simulink model "check_other_Potential"  (R2023b)
settings: Solver=ode5  StartTime=0.0  StopTime=2  FixedStep=0.0001  RelTol=1e-3
settings Model: Creator=amaiani  LastModifiedBy=amaiani

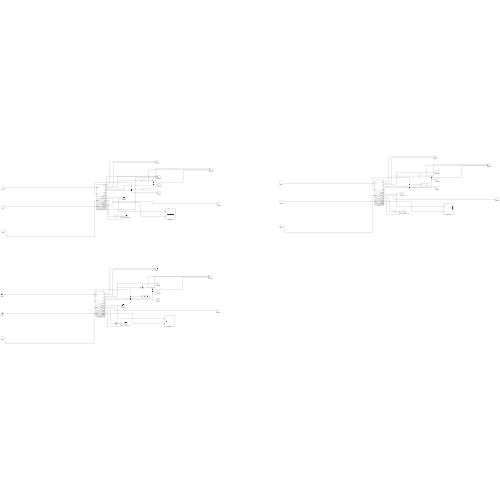
[thumbnail: Simulink's stored preview of the top-level diagram]
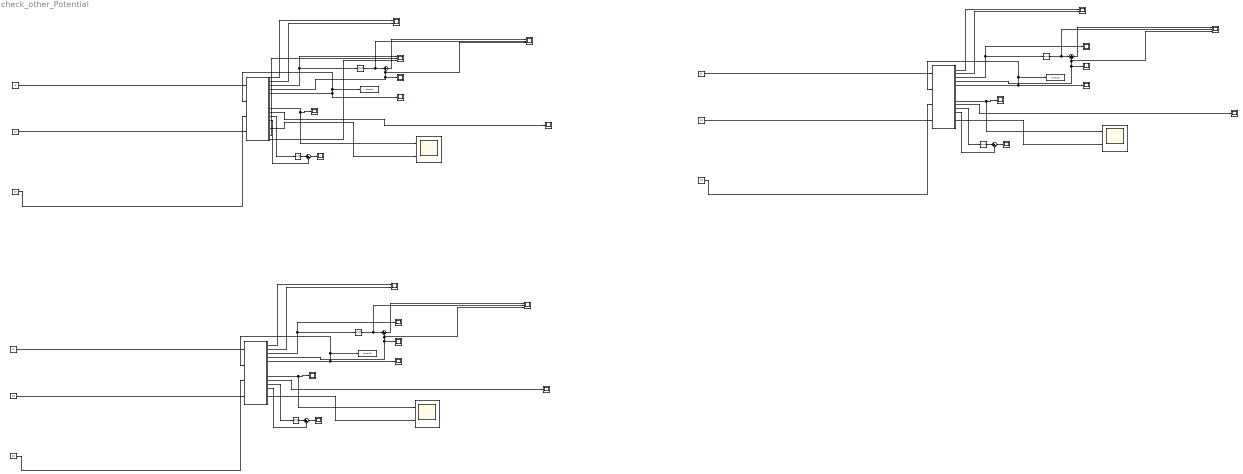
== system check_other_Potential ==
  Damp : Constant  Value=10
  Damp1 : Constant  Value=10
  Damp2 : Constant  Value=10
  Derivative{,1..5} (6 alike) : Derivative
  Dynamics{,1..5} (6 alike) : Scope
  H_dot_error : Scope  NumInputPorts=3
  H_dot_error1 : Scope  NumInputPorts=3
  H_dot_error2 : Scope  NumInputPorts=3
  H_dot_theory : Scope
  H_dot_theory1 : Scope
  H_dot_theory2 : Scope
  Hamiltonian : Scope  NumInputPorts=3
  Hamiltonian1 : Scope
  Hamiltonian2 : Scope
  Liu : Subsystem
  Liu1 : Subsystem
  Liu2 : Subsystem
  Sum{,1..5} (6 alike) : Sum  Inputs=|+-
  To Workspace : ToWorkspace  VariableName=simout  SampleTime=-1
  To Workspace1 : ToWorkspace  VariableName=simout1  SampleTime=-1
  To Workspace2 : ToWorkspace  VariableName=simout2  SampleTime=-1
  added_power : Scope  NumInputPorts=2
  added_power1 : Scope  NumInputPorts=2
  added_power2 : Scope  NumInputPorts=2
  alpha : Constant  Value=10
  alpha1 : Constant  Value=10
  alpha2 : Constant  Value=10
  cbf_dot_measured_error : Scope
  cbf_dot_measured_error1 : Scope
  cbf_dot_measured_error2 : Scope
  dhdqqdot : Scope
  dhdqqdot1 : Scope
  dhdqqdot2 : Scope
  skew : Scope  NumInputPorts=2
  skew1 : Scope  NumInputPorts=2
  skew2 : Scope  NumInputPorts=2
  spring : Constant  Value=[10,0,0;0,1,0;0,0,1]
  spring1 : Constant  Value=[10,0,0;0,10,0;0,0,10]
  spring2 : Constant  Value=[10,0,0;0,1,0;0,0,1]
  wires:
  Derivative/1 -> H_dot_error/2, Sum/1
  Sum/1 -> H_dot_error/1
  spring/1 -> Liu/1(spring)
  Damp/1 -> Liu/4(damp)
  alpha/1 -> Liu/3(alpha)
  Liu/4(H_dot) -> H_dot_theory/1, H_dot_error/3, Sum/2
  Liu/5(Out5) -> Dynamics/1, Liu/2(q), To Workspace/1
  Liu/3(E) -> Derivative/1, Hamiltonian/1
  Liu/1(out_1) -> skew/1
  Liu/2(out_2) -> skew/2
  Liu/10(hessian_term) -> Dynamics1/1
  Liu/9(before_dot) -> added_power/1, dhdqqdot/1
  Liu/11(cbf) -> Derivative1/1
  Derivative1/1 -> Sum2/1
  Sum2/1 -> cbf_dot_measured_error/1
  Liu/12(cbf_dot) -> Sum2/2
  Liu/14(after_dot) -> added_power/2
  Damp1/1 -> Liu1/4(damp)
  Liu1/2(out_2) -> skew1/2
  Liu1/11(cbf) -> Derivative3/1
  spring1/1 -> Liu1/1(spring)
  alpha1/1 -> Liu1/3(alpha)
  Liu1/5(Out5) -> Dynamics2/1, Liu1/2(q), To Workspace1/1
  Sum3/1 -> cbf_dot_measured_error1/1
  Liu1/1(out_1) -> skew1/1
  Liu1/10(hessian_term) -> Dynamics3/1
  Derivative2/1 -> H_dot_error1/2, Sum1/1
  Liu1/3(E) -> Derivative2/1, Hamiltonian1/1
  Derivative3/1 -> Sum3/1
  Liu1/12(cbf_dot) -> Sum3/2
  Sum1/1 -> H_dot_error1/1
  Liu1/4(H_dot) -> H_dot_theory1/1, H_dot_error1/3, Sum1/2
  Liu1/14(after_dot) -> added_power1/2
  Liu1/9(before_dot) -> added_power1/1, dhdqqdot1/1
  Damp2/1 -> Liu2/4(damp)
  Liu2/2(out_2) -> skew2/2
  Liu2/11(cbf) -> Derivative5/1
  spring2/1 -> Liu2/1(spring)
  alpha2/1 -> Liu2/3(alpha)
  Liu2/5(Out5) -> Dynamics4/1, Liu2/2(q), To Workspace2/1
  Sum5/1 -> cbf_dot_measured_error2/1
  Liu2/1(out_1) -> skew2/1
  Liu2/10(hessian_term) -> Dynamics5/1
  Derivative4/1 -> H_dot_error2/2, Sum4/1
  Liu2/3(E) -> Derivative4/1, Hamiltonian2/1
  Derivative5/1 -> Sum5/1
  Liu2/12(cbf_dot) -> Sum5/2
  Sum4/1 -> H_dot_error2/1
  Liu2/4(H_dot) -> H_dot_theory2/1, H_dot_error2/3, Sum4/2
  Liu2/14(after_dot) -> added_power2/2
  Liu2/9(before_dot) -> added_power2/1, dhdqqdot2/1
  Liu/16(T) -> Hamiltonian/2
  Liu/17(V) -> Hamiltonian/3

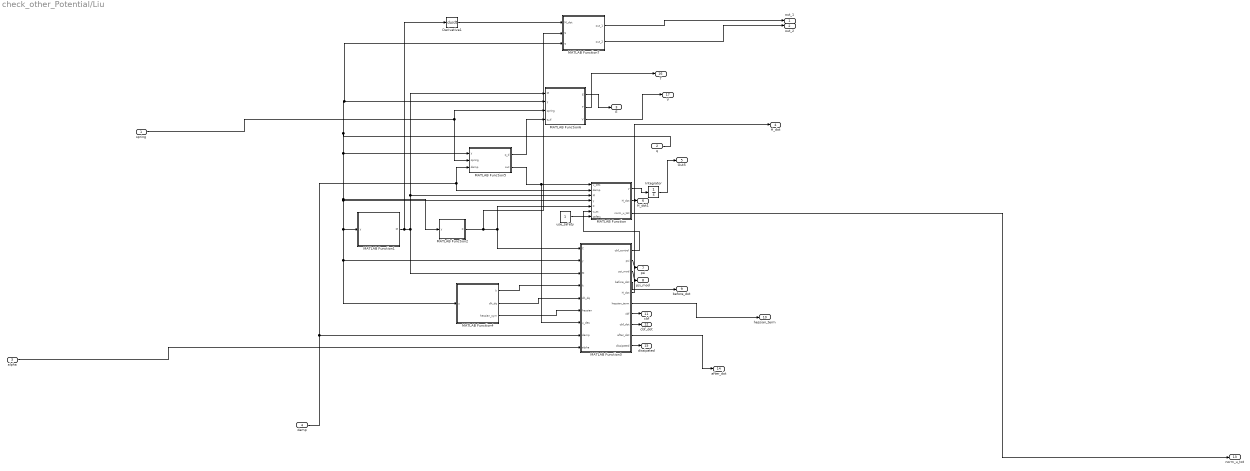
== system check_other_Potential/Liu ==
  spring : Inport
  q : Inport  Port=2
  alpha : Inport  Port=3
  damp : Inport  Port=4
  Derivative1 : Derivative
  Integrator : Integrator  InitialCondition=[0;0;0;0;0;0]
  MATLAB Function : MATLAB Function  TreatAsAtomicUnit=on
  MATLAB Function1 : MATLAB Function  StartFcn=|  TreatAsAtomicUnit=on
      | % Define numerical values for the parameters
      | xc = 2.5;
      | yc = 2;
      | r = 1;
      | gamma = 2;
      | alpha = 20;
      | 
      | 
      | m1 = 1;
      | m2 = 1;
      | m3 = 1;
      | 
      | 
      | l1 = 1;
      | l2 = 1;
      | l3 = 1;
  MATLAB Function2 : MATLAB Function  StartFcn=|  TreatAsAtomicUnit=on
      | % Define numerical values for the parameters
      | xc = 2.5;
      | yc = 2;
      | r = 1;
      | gamma = 2;
      | alpha = 20;
      | 
      | 
      | m1 = 1;
      | m2 = 1;
      | m3 = 1;
      | 
      | 
      | l1 = 1;
      | l2 = 1;
      | l3 = 1;
  MATLAB Function3 : MATLAB Function  TreatAsAtomicUnit=on
  MATLAB Function4 : MATLAB Function  TreatAsAtomicUnit=on
  MATLAB Function5 : MATLAB Function  TreatAsAtomicUnit=on
  MATLAB Function6 : MATLAB Function  TreatAsAtomicUnit=on
  MATLAB Function7 : MATLAB Function  StartFcn=|  TreatAsAtomicUnit=on
      | % Define numerical values for the parameters
      | xc = 2.5;
      | yc = 2;
      | r = 1;
      | gamma = 2;
      | alpha = 20;
      | 
      | 
      | m1 = 1;
      | m2 = 1;
      | m3 = 1;
      | 
      | 
      | l1 = 1;
      | l2 = 1;
      | l3 = 1;
  use_safety : Constant
  out_1 : Outport
  out_2 : Outport  Port=2
  E : Outport  Port=3
  H_dot : Outport  Port=4
  Out5 : Outport  Port=5
  H_dot1 : Outport  Port=6
  psi : Outport  Port=7
  psi_mod : Outport  Port=8
  before_dot : Outport  Port=9
  hessian_term : Outport  Port=10
  cbf : Outport  Port=11
  cbf_dot : Outport  Port=12
  norm_u_tot : Outport  Port=13
  after_dot : Outport  Port=14
  dissipated : Outport  Port=15
  T : Outport  Port=16
  V : Outport  Port=17
  wires:
  MATLAB Function3/8(cbf_dot) -> cbf_dot/1
  MATLAB Function3/2(psi) -> psi/1
  MATLAB Function3/7(cbf) -> cbf/1
  MATLAB Function/3(norm_u_tot) -> norm_u_tot/1
  MATLAB Function/2(H_dot) -> H_dot1/1
  Integrator/1 -> Out5/1
  MATLAB Function4/3(hessian_sym) -> MATLAB Function3/6(hessian)
  MATLAB Function1/1(M) -> Derivative1/1, MATLAB Function6/1(M), MATLAB Function/3(M), MATLAB Function3/3(M)
  MATLAB Function4/2(dh_dq) -> MATLAB Function3/5(dh_dq)
  MATLAB Function7/1(out_1) -> out_1/1
  alpha/1 -> MATLAB Function3/9(alpha)
  MATLAB Function6/1(E) -> E/1
  MATLAB Function3/3(psi_mod) -> psi_mod/1
  MATLAB Function7/2(out_2) -> out_2/1
  use_safety/1 -> MATLAB Function/7(safety)
  MATLAB Function3/4(before_dot) -> before_dot/1
  Derivative1/1 -> MATLAB Function7/1(M_dot)
  MATLAB Function5/1(q_d) -> MATLAB Function6/4(q_d)
  MATLAB Function3/5(H_dot) -> H_dot/1
  MATLAB Function/1(y) -> Integrator/1
  MATLAB Function3/1(cbf_control) -> MATLAB Function/6(u_sc)
  MATLAB Function2/1(C) -> MATLAB Function/5(C), MATLAB Function3/1(C), MATLAB Function7/2(S)
  MATLAB Function4/1(h) -> MATLAB Function3/4(h)
  spring/1 -> MATLAB Function6/3(spring), MATLAB Function5/2(spring)
  MATLAB Function5/2(out) -> MATLAB Function3/7(u_des), MATLAB Function/1(u_des)
  MATLAB Function3/6(hessian_term) -> hessian_term/1
  q/1 -> MATLAB Function7/3(q), MATLAB Function6/2(y), MATLAB Function5/1(y), MATLAB Function2/1(y), MATLAB Function4/1(y), MATLAB Function3/2(y), MATLAB Function1/1(y), MATLAB Function/4("y ")
  damp/1 -> MATLAB Function/2(damp), MATLAB Function5/3(damp), MATLAB Function3/8(damp)
  MATLAB Function3/9(after_dot) -> after_dot/1
  MATLAB Function3/10(dissipated) -> dissipated/1
  MATLAB Function6/2(T) -> T/1
  MATLAB Function6/3(V) -> V/1

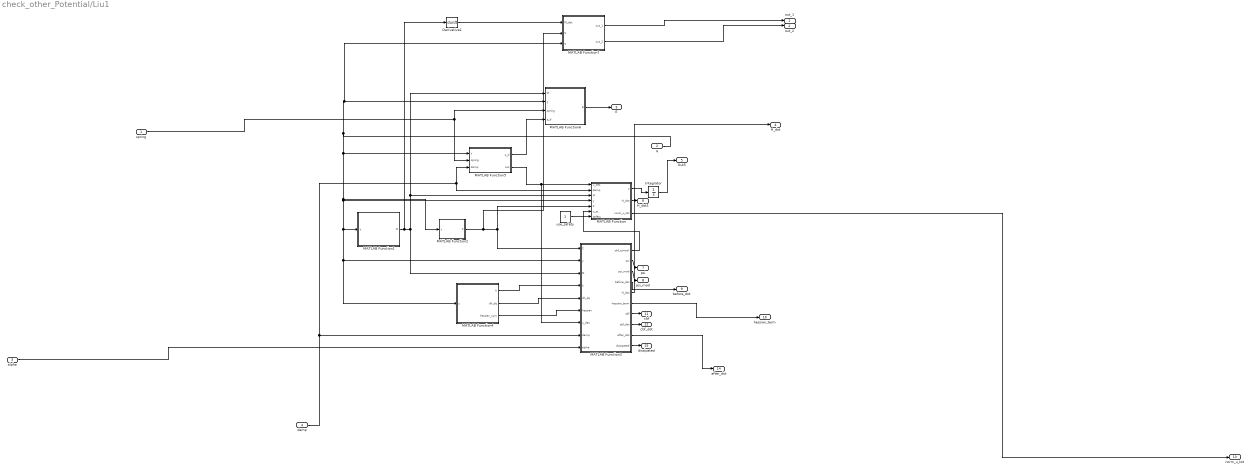
== system check_other_Potential/Liu1 ==
  spring : Inport
  q : Inport  Port=2
  alpha : Inport  Port=3
  damp : Inport  Port=4
  Derivative1 : Derivative
  Integrator : Integrator  InitialCondition=[0;0;0;0;0;0]
  MATLAB Function : MATLAB Function  TreatAsAtomicUnit=on
  MATLAB Function1 : MATLAB Function  StartFcn=|  TreatAsAtomicUnit=on
      | % Define numerical values for the parameters
      | xc = 2.5;
      | yc = 2;
      | r = 1;
      | gamma = 2;
      | alpha = 20;
      | 
      | 
      | m1 = 1;
      | m2 = 1;
      | m3 = 1;
      | 
      | 
      | l1 = 1;
      | l2 = 1;
      | l3 = 1;
  MATLAB Function2 : MATLAB Function  StartFcn=|  TreatAsAtomicUnit=on
      | % Define numerical values for the parameters
      | xc = 2.5;
      | yc = 2;
      | r = 1;
      | gamma = 2;
      | alpha = 20;
      | 
      | 
      | m1 = 1;
      | m2 = 1;
      | m3 = 1;
      | 
      | 
      | l1 = 1;
      | l2 = 1;
      | l3 = 1;
  MATLAB Function3 : MATLAB Function  TreatAsAtomicUnit=on
  MATLAB Function4 : MATLAB Function  TreatAsAtomicUnit=on
  MATLAB Function5 : MATLAB Function  TreatAsAtomicUnit=on
  MATLAB Function6 : MATLAB Function  TreatAsAtomicUnit=on
  MATLAB Function7 : MATLAB Function  StartFcn=|  TreatAsAtomicUnit=on
      | % Define numerical values for the parameters
      | xc = 2.5;
      | yc = 2;
      | r = 1;
      | gamma = 2;
      | alpha = 20;
      | 
      | 
      | m1 = 1;
      | m2 = 1;
      | m3 = 1;
      | 
      | 
      | l1 = 1;
      | l2 = 1;
      | l3 = 1;
  use_safety : Constant
  out_1 : Outport
  out_2 : Outport  Port=2
  E : Outport  Port=3
  H_dot : Outport  Port=4
  Out5 : Outport  Port=5
  H_dot1 : Outport  Port=6
  psi : Outport  Port=7
  psi_mod : Outport  Port=8
  before_dot : Outport  Port=9
  hessian_term : Outport  Port=10
  cbf : Outport  Port=11
  cbf_dot : Outport  Port=12
  norm_u_tot : Outport  Port=13
  after_dot : Outport  Port=14
  dissipated : Outport  Port=15
  wires:
  MATLAB Function3/8(cbf_dot) -> cbf_dot/1
  MATLAB Function3/2(psi) -> psi/1
  MATLAB Function3/7(cbf) -> cbf/1
  MATLAB Function/3(norm_u_tot) -> norm_u_tot/1
  MATLAB Function/2(H_dot) -> H_dot1/1
  Integrator/1 -> Out5/1
  MATLAB Function4/3(hessian_sym) -> MATLAB Function3/6(hessian)
  MATLAB Function1/1(M) -> Derivative1/1, MATLAB Function6/1(M), MATLAB Function/3(M), MATLAB Function3/3(M)
  MATLAB Function4/2(dh_dq) -> MATLAB Function3/5(dh_dq)
  MATLAB Function7/1(out_1) -> out_1/1
  alpha/1 -> MATLAB Function3/9(alpha)
  MATLAB Function6/1(E) -> E/1
  MATLAB Function3/3(psi_mod) -> psi_mod/1
  MATLAB Function7/2(out_2) -> out_2/1
  use_safety/1 -> MATLAB Function/7(safety)
  MATLAB Function3/4(before_dot) -> before_dot/1
  Derivative1/1 -> MATLAB Function7/1(M_dot)
  MATLAB Function5/1(q_d) -> MATLAB Function6/4(q_d)
  MATLAB Function3/5(H_dot) -> H_dot/1
  MATLAB Function/1(y) -> Integrator/1
  MATLAB Function3/1(cbf_control) -> MATLAB Function/6(u_sc)
  MATLAB Function2/1(C) -> MATLAB Function/5(C), MATLAB Function3/1(C), MATLAB Function7/2(S)
  MATLAB Function4/1(h) -> MATLAB Function3/4(h)
  spring/1 -> MATLAB Function6/3(spring), MATLAB Function5/2(spring)
  MATLAB Function5/2(out) -> MATLAB Function3/7(u_des), MATLAB Function/1(u_des)
  MATLAB Function3/6(hessian_term) -> hessian_term/1
  q/1 -> MATLAB Function7/3(q), MATLAB Function6/2(y), MATLAB Function5/1(y), MATLAB Function2/1(y), MATLAB Function4/1(y), MATLAB Function3/2(y), MATLAB Function1/1(y), MATLAB Function/4("y ")
  damp/1 -> MATLAB Function/2(damp), MATLAB Function5/3(damp), MATLAB Function3/8(damp)
  MATLAB Function3/9(after_dot) -> after_dot/1
  MATLAB Function3/10(dissipated) -> dissipated/1

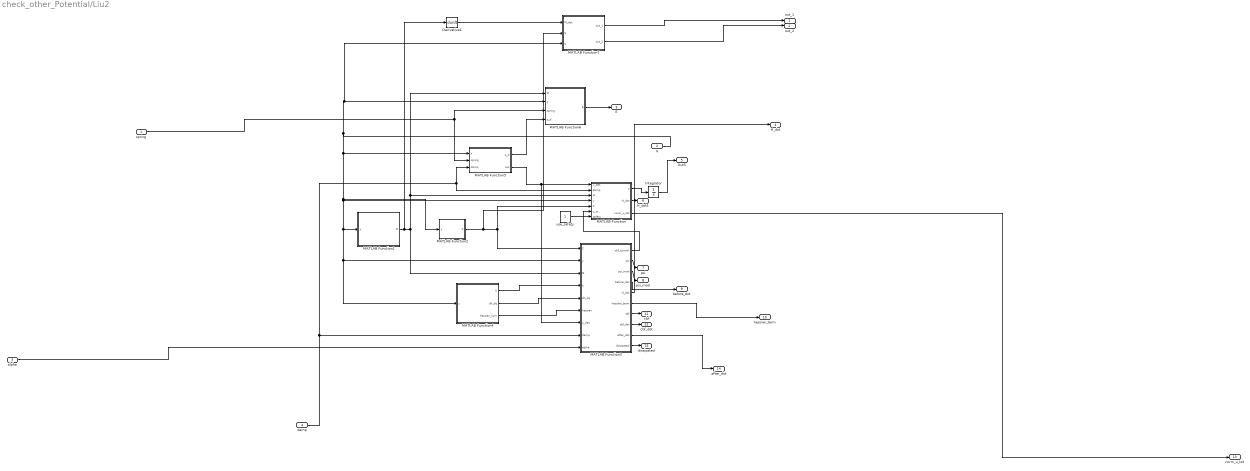
== system check_other_Potential/Liu2 ==
  spring : Inport
  q : Inport  Port=2
  alpha : Inport  Port=3
  damp : Inport  Port=4
  Derivative1 : Derivative
  Integrator : Integrator  InitialCondition=[0;0;0;0;0;0]
  MATLAB Function : MATLAB Function  TreatAsAtomicUnit=on
  MATLAB Function1 : MATLAB Function  StartFcn=|  TreatAsAtomicUnit=on
      | % Define numerical values for the parameters
      | xc = 2.5;
      | yc = 2;
      | r = 1;
      | gamma = 2;
      | alpha = 20;
      | 
      | 
      | m1 = 1;
      | m2 = 1;
      | m3 = 1;
      | 
      | 
      | l1 = 1;
      | l2 = 1;
      | l3 = 1;
  MATLAB Function2 : MATLAB Function  StartFcn=|  TreatAsAtomicUnit=on
      | % Define numerical values for the parameters
      | xc = 2.5;
      | yc = 2;
      | r = 1;
      | gamma = 2;
      | alpha = 20;
      | 
      | 
      | m1 = 1;
      | m2 = 1;
      | m3 = 1;
      | 
      | 
      | l1 = 1;
      | l2 = 1;
      | l3 = 1;
  MATLAB Function3 : MATLAB Function  TreatAsAtomicUnit=on
  MATLAB Function4 : MATLAB Function  TreatAsAtomicUnit=on
  MATLAB Function5 : MATLAB Function  TreatAsAtomicUnit=on
  MATLAB Function6 : MATLAB Function  TreatAsAtomicUnit=on
  MATLAB Function7 : MATLAB Function  StartFcn=|  TreatAsAtomicUnit=on
      | % Define numerical values for the parameters
      | xc = 2.5;
      | yc = 2;
      | r = 1;
      | gamma = 2;
      | alpha = 20;
      | 
      | 
      | m1 = 1;
      | m2 = 1;
      | m3 = 1;
      | 
      | 
      | l1 = 1;
      | l2 = 1;
      | l3 = 1;
  use_safety : Constant
  out_1 : Outport
  out_2 : Outport  Port=2
  E : Outport  Port=3
  H_dot : Outport  Port=4
  Out5 : Outport  Port=5
  H_dot1 : Outport  Port=6
  psi : Outport  Port=7
  psi_mod : Outport  Port=8
  before_dot : Outport  Port=9
  hessian_term : Outport  Port=10
  cbf : Outport  Port=11
  cbf_dot : Outport  Port=12
  norm_u_tot : Outport  Port=13
  after_dot : Outport  Port=14
  dissipated : Outport  Port=15
  wires:
  MATLAB Function3/8(cbf_dot) -> cbf_dot/1
  MATLAB Function3/2(psi) -> psi/1
  MATLAB Function3/7(cbf) -> cbf/1
  MATLAB Function/3(norm_u_tot) -> norm_u_tot/1
  MATLAB Function/2(H_dot) -> H_dot1/1
  Integrator/1 -> Out5/1
  MATLAB Function4/3(hessian_sym) -> MATLAB Function3/6(hessian)
  MATLAB Function1/1(M) -> Derivative1/1, MATLAB Function6/1(M), MATLAB Function/3(M), MATLAB Function3/3(M)
  MATLAB Function4/2(dh_dq) -> MATLAB Function3/5(dh_dq)
  MATLAB Function7/1(out_1) -> out_1/1
  alpha/1 -> MATLAB Function3/9(alpha)
  MATLAB Function6/1(E) -> E/1
  MATLAB Function3/3(psi_mod) -> psi_mod/1
  MATLAB Function7/2(out_2) -> out_2/1
  use_safety/1 -> MATLAB Function/7(safety)
  MATLAB Function3/4(before_dot) -> before_dot/1
  Derivative1/1 -> MATLAB Function7/1(M_dot)
  MATLAB Function5/1(q_d) -> MATLAB Function6/4(q_d)
  MATLAB Function3/5(H_dot) -> H_dot/1
  MATLAB Function/1(y) -> Integrator/1
  MATLAB Function3/1(cbf_control) -> MATLAB Function/6(u_sc)
  MATLAB Function2/1(C) -> MATLAB Function/5(C), MATLAB Function3/1(C), MATLAB Function7/2(S)
  MATLAB Function4/1(h) -> MATLAB Function3/4(h)
  spring/1 -> MATLAB Function6/3(spring), MATLAB Function5/2(spring)
  MATLAB Function5/2(out) -> MATLAB Function3/7(u_des), MATLAB Function/1(u_des)
  MATLAB Function3/6(hessian_term) -> hessian_term/1
  q/1 -> MATLAB Function7/3(q), MATLAB Function6/2(y), MATLAB Function5/1(y), MATLAB Function2/1(y), MATLAB Function4/1(y), MATLAB Function3/2(y), MATLAB Function1/1(y), MATLAB Function/4("y ")
  damp/1 -> MATLAB Function/2(damp), MATLAB Function5/3(damp), MATLAB Function3/8(damp)
  MATLAB Function3/9(after_dot) -> after_dot/1
  MATLAB Function3/10(dissipated) -> dissipated/1

== matlab function check_other_Potential/Liu/MATLAB Function6 ==
  data: M input; E output; y input; spring input; q_d input; T output; V output
function [E,T,V] = energy(M,y,spring, q_d)
    q = y(1:3);
    dq = y(4:6);
    T = 0.5 * (dq' * M * dq);
    V = 0.5 * (q-q_d)' *spring* (q-q_d);
    E = T + V;

== matlab function check_other_Potential/Liu/MATLAB Function7 ==
  data: M_dot input; out_1 output; S input; q input; out_2 output


function [out_1, out_2] = M_dot_coriolis_check(M_dot,S, q)
    dq = reshape(q(4:6),[3,1]);
    
    q1 = q(1);
    q2 = q(2);
    q3 = q(3);
    dq1 = q(4);
    dq2 = q(5);
    dq3 = q(6);

    check = M_dot - 2 * S;


    out_1 = dq' * check * dq;


    M_dot_formula =   [        - dq2*(sin(q2 + q3) + 3*sin(q2)) - dq3*(sin(q2 + q3) + sin(q3)), - dq3*(sin(q2 + q3)/2 + sin(q3)) - dq2*(sin(q2 + q3)/2 + (3*sin(q2))/2), - (dq2*sin(q2 + q3))/2 - dq3*(sin(q2 + q3)/2 + sin(q3)/2);
- dq3*(sin(q2 + q3)/2 + sin(q3)) - dq2*(sin(q2 + q3)/2 + (3*sin(q2))/2),                                                            -dq3*sin(q3),                                          -(dq3*sin(q3))/2;
              - (dq2*sin(q2 + q3))/2 - dq3*(sin(q2 + q3)/2 + sin(q3)/2),                                                        -(dq3*sin(q3))/2,                                                         0];
 

    
    out_2 = dq' * (M_dot_formula - 2 * S) * dq;
end

== matlab function check_other_Potential/Liu1/MATLAB Function ==
  data: u_des input; damp input; M input; y input; y output; C input; H_dot output; u_sc input; safety input; norm_u_tot output
function [y,H_dot,norm_u_tot]= dynamics(u_des, damp , M,y, C, u_sc, safety)
    
    q = reshape(y(1:3),[3,1]);
    dq = reshape(y(4:6),[3,1]);



    [~, p] = chol(M);
    decision = (p == 0);

    assert(decision, 'Inertia matrix is not positive definite');
    
    u_tot = u_des + safety * u_sc;
    norm_u_tot=norm(u_tot);
    ddq = inv(M) * (u_tot - C * dq ); % + u_sc

    H_dot = - dq' * damp * dq;

    y = [dq; ddq];

== matlab function check_other_Potential/Liu1/MATLAB Function1 ==
  data: y input; M output
function M = inertia_M(y)

    q1 = y(1);
    q2 = y(2);
    q3 = y(3);

    M  = [        cos(q2 + q3) + 3*cos(q2) + cos(q3) + 4, cos(q2 + q3)/2 + (3*cos(q2))/2 + cos(q3) + 5/3, cos(q2 + q3)/2 + cos(q3)/2 + 1/3;
cos(q2 + q3)/2 + (3*cos(q2))/2 + cos(q3) + 5/3,                                  cos(q3) + 5/3,                  cos(q3)/2 + 1/3;
              cos(q2 + q3)/2 + cos(q3)/2 + 1/3,                                cos(q3)/2 + 1/3,                              1/3];

    assert(isequal(M, M'),'error')

== matlab function check_other_Potential/Liu1/MATLAB Function2 ==
  data: y input; C output
function C = coriolis(y)

    q1 = y(1);
    q2 = y(2);
    q3 = y(3);
    dq1 = y(4);
    dq2 = y(5);
    dq3 = y(6);


    C = [- dq2*(sin(q2 + q3)/2 + (3*sin(q2))/2) - dq3*(sin(q2 + q3)/2 + sin(q3)/2), - dq1*(sin(q2 + q3)/2 + (3*sin(q2))/2) - dq2*(sin(q2 + q3)/2 + (3*sin(q2))/2) - dq3*(sin(q2 + q3)/2 + sin(q3)/2), - dq1*(sin(q2 + q3)/2 + sin(q3)/2) - dq2*(sin(q2 + q3)/2 + sin(q3)/2) - dq3*(sin(q2 + q3)/2 + sin(q3)/2);
                dq1*(sin(q2 + q3)/2 + (3*sin(q2))/2) - (dq3*sin(q3))/2,                                                                                                 -(dq3*sin(q3))/2,                                                    - (dq1*sin(q3))/2 - (dq2*sin(q3))/2 - (dq3*sin(q3))/2;
                       dq1*(sin(q2 + q3)/2 + sin(q3)/2) + (dq2*sin(q3))/2,                                                                                (dq1*sin(q3))/2 + (dq2*sin(q3))/2,                                                                                                        0];

== matlab function check_other_Potential/Liu1/MATLAB Function3 ==
  data: C input; y input; cbf_control output; M input; h input; dh_dq input; hessian input; u_des input; psi output; psi_mod output; before_dot output; H_dot output; damp input; hessian_term output; cbf output; cbf_dot output; alpha input; after_dot output; dissipated output

function [cbf_control, psi, psi_mod,before_dot, H_dot, hessian_term, cbf, cbf_dot, after_dot, dissipated]= CBF(C, y, M, h, dh_dq, hessian, u_des, damp, alpha)
% Define numerical values for the parameters
    xc = 2.5;
    yc = 2;
    r = 1;
    gamma = 2;

    
    m1 = 1;
    m2 = 1;
    m3 = 1;
    
    l1 = 1;
    l2 = 1;
    l3 = 1;
    
    q = reshape(y(1:3),[3,1]);
    dq = reshape(y(4:6),[3,1]);
    dh_dq = reshape(dh_dq,[1,3]);

    LIU = 1;

    M_inv = inv(M);

    before_dot = dh_dq * dq;
    after_dot = dh_dq * M_inv * dq;



    d = eig(M_inv);
    tol = 10^(-5);
    check = all(abs(M_inv - M_inv') < tol, 'all');
    assert(check,'error')
    % assert(isequal(M_inv, M_inv'),'error')

    assert(all(d>0),'error_m_inv')

    active = 0;

    if LIU == 1

    
        cbf = alpha * h + dh_dq * dq;
        lg_h = zeros(1,3);
        cbf_dot_prior = alpha .* dh_dq * dq + dq' * hessian * dq + dh_dq * (M_inv* (-C * dq + u_des));
        psi = cbf_dot_prior + gamma .* cbf;
        if psi<0
            lg_h = dh_dq * M_inv;
            
            cbf_control =  - lg_h' /(lg_h * lg_h')  .* psi;
            active = 1;
        else
            cbf_control = zeros(3,1);

        end
        cbf_dot = alpha .* dh_dq * dq + dq' * hessian * dq + dh_dq * M_inv* (-C * dq + u_des+ cbf_control);
        psi_mod = cbf_dot + gamma .* cbf;

        H_dot = dq' * cbf_control - dq' * damp * dq;
        
        dissipated= - dq' * damp * dq;

        hessian_term = dq' * hessian * dq;
        
    
    else
        KE = 0.5 * dq' * M * dq;
        cbf = alpha * h - KE;
        lg_h = zeros(1,3);
        cbf_dot_prior = alpha .* dh_dq * dq - dq' * M_inv * u_des;
        psi = cbf_dot_prior + gamma .* cbf;
        if psi<0
            lg_h = -dq';
            cbf_control =  dq /(dq'*dq)  .* psi;
        else
            cbf_control = zeros(3,1);
        end
        cbf_dot =  alpha .* dh_dq * dq - dq' * M_inv * (u_des+cbf_control) ;
        psi_mod = cbf_dot + gamma .* cbf;

        H_dot = dq' * cbf_control - dq' * damp * dq;


        hessian_term = 0;
 
        
    end
    
end

== matlab function check_other_Potential/Liu1/MATLAB Function4 ==
  data: y input; h output; dh_dq output; hessian_sym output
function [h, dh_dq, hessian_sym] = obstacle(y)
    % Define numerical values for the parameters
    xc = 2.5;
    yc = 2;
    r = 1;

    l1 = 1;
    l2 = 1;
    l3 = 1;
    
    % Compute the end-effector position using forward kinematics
    q1 = y(1);
    q2 = y(2);
    q3 = y(3);
    
    x_ee = l1 * cos(q1) + l2 * cos(q1 + q2) + l3 * cos(q1 + q2 + q3);
    y_ee = l1 * sin(q1) + l2 * sin(q1 + q2) + l3 * sin(q1 + q2 + q3);
    
    % Compute the control barrier function h
    h = (xc - x_ee)^2 + (yc - y_ee)^2 - r^2;
    
    % Define the expressions for dh_dq and hessian_sym
    dh_dq = [2*(cos(q1 + q2 + q3) + cos(q1 + q2) + cos(q1))*(sin(q1 + q2 + q3) + sin(q1 + q2) + sin(q1) - 2) - 2*(sin(q1 + q2 + q3) + sin(q1 + q2) + sin(q1))*(cos(q1 + q2 + q3) + cos(q1 + q2) + cos(q1) - 5/2), 2*(cos(q1 + q2 + q3) + cos(q1 + q2))*(sin(q1 + q2 + q3) + sin(q1 + q2) + sin(q1) - 2) - 2*(sin(q1 + q2 + q3) + sin(q1 + q2))*(cos(q1 + q2 + q3) + cos(q1 + q2) + cos(q1) - 5/2), 2*cos(q1 + q2 + q3)*(sin(q1 + q2 + q3) + sin(q1 + q2) + sin(q1) - 2) - 2*sin(q1 + q2 + q3)*(cos(q1 + q2 + q3) + cos(q1 + q2) + cos(q1) - 5/2)];


    hessian_sym = [                                              2*(cos(q1 + q2 + q3) + cos(q1 + q2) + cos(q1))^2 - 2*(cos(q1 + q2 + q3) + cos(q1 + q2) + cos(q1))*(cos(q1 + q2 + q3) + cos(q1 + q2) + cos(q1) - 5/2) + 2*(sin(q1 + q2 + q3) + sin(q1 + q2) + sin(q1))^2 - 2*(sin(q1 + q2 + q3) + sin(q1 + q2) + sin(q1))*(sin(q1 + q2 + q3) + sin(q1 + q2) + sin(q1) - 2), 2*(cos(q1 + q2 + q3) + cos(q1 + q2))*(cos(q1 + q2 + q3) + cos(q1 + q2) + cos(q1)) - 2*(cos(q1 + q2 + q3) + cos(q1 + q2))*(cos(q1 + q2 + q3) + cos(q1 + q2) + cos(q1) - 5/2) + 2*(sin(q1 + q2 + q3) + sin(q1 + q2))*(sin(q1 + q2 + q3) + sin(q1 + q2) + sin(q1)) - 2*(sin(q1 + q2 + q3) + sin(q1 + q2))*(sin(q1 + q2 + q3) + sin(q1 + q2) + sin(q1) - 2), 2*cos(q1 + q2 + q3)*(cos(q1 + q2 + q3) + cos(q1 + q2) + cos(q1)) - 2*cos(q1 + q2 + q3)*(cos(q1 + q2 + q3) + cos(q1 + q2) + cos(q1) - 5/2) + 2*sin(q1 + q2 + q3)*(sin(q1 + q2 + q3) + sin(q1 + q2) + sin(q1)) - 2*sin(q1 + q2 + q3)*(sin(q1 + q2 + q3) + sin(q1 + q2) + sin(q1) - 2);
        2*(cos(q1 + q2 + q3) + cos(q1 + q2))*(cos(q1 + q2 + q3) + cos(q1 + q2) + cos(q1)) - 2*(cos(q1 + q2 + q3) + cos(q1 + q2))*(cos(q1 + q2 + q3) + cos(q1 + q2) + cos(q1) - 5/2) + 2*(sin(q1 + q2 + q3) + sin(q1 + q2))*(sin(q1 + q2 + q3) + sin(q1 + q2) + sin(q1)) - 2*(sin(q1 + q2 + q3) + sin(q1 + q2))*(sin(q1 + q2 + q3) + sin(q1 + q2) + sin(q1) - 2),                                                                                       2*(cos(q1 + q2 + q3) + cos(q1 + q2))^2 - 2*(cos(q1 + q2 + q3) + cos(q1 + q2))*(cos(q1 + q2 + q3) + cos(q1 + q2) + cos(q1) - 5/2) + 2*(sin(q1 + q2 + q3) + sin(q1 + q2))^2 - 2*(sin(q1 + q2 + q3) + sin(q1 + q2))*(sin(q1 + q2 + q3) + sin(q1 + q2) + sin(q1) - 2),                     2*cos(q1 + q2 + q3)*(cos(q1 + q2 + q3) + cos(q1 + q2)) - 2*cos(q1 + q2 + q3)*(cos(q1 + q2 + q3) + cos(q1 + q2) + cos(q1) - 5/2) - 2*sin(q1 + q2 + q3)*(sin(q1 + q2 + q3) + sin(q1 + q2) + sin(q1) - 2) + 2*sin(q1 + q2 + q3)*(sin(q1 + q2 + q3) + sin(q1 + q2));
                                                                            2*cos(q1 + q2 + q3)*(cos(q1 + q2 + q3) + cos(q1 + q2) + cos(q1)) - 2*cos(q1 + q2 + q3)*(cos(q1 + q2 + q3) + cos(q1 + q2) + cos(q1) - 5/2) + 2*sin(q1 + q2 + q3)*(sin(q1 + q2 + q3) + sin(q1 + q2) + sin(q1)) - 2*sin(q1 + q2 + q3)*(sin(q1 + q2 + q3) + sin(q1 + q2) + sin(q1) - 2),                                                                                         2*cos(q1 + q2 + q3)*(cos(q1 + q2 + q3) + cos(q1 + q2)) - 2*cos(q1 + q2 + q3)*(cos(q1 + q2 + q3) + cos(q1 + q2) + cos(q1) - 5/2) - 2*sin(q1 + q2 + q3)*(sin(q1 + q2 + q3) + sin(q1 + q2) + sin(q1) - 2) + 2*sin(q1 + q2 + q3)*(sin(q1 + q2 + q3) + sin(q1 + q2)),                                                                                       2*cos(q1 + q2 + q3)^2 - 2*cos(q1 + q2 + q3)*(cos(q1 + q2 + q3) + cos(q1 + q2) + cos(q1) - 5/2) + 2*sin(q1 + q2 + q3)^2 - 2*sin(q1 + q2 + q3)*(sin(q1 + q2 + q3) + sin(q1 + q2) + sin(q1) - 2)];
     

    % d = eig(hessian_sym)
    % isposdef = all(d >= 0);
    % 
    % assert(isposdef, 'error hessian');
end

== matlab function check_other_Potential/Liu1/MATLAB Function5 ==
  data: q_d output; y input; spring input; out output; damp input
function [q_d, out] = u_des(y, spring, damp)


    q = reshape(y(1:3),[3,1]);
    dq = reshape(y(4:6),[3,1]);

    q_d = [pi; 0; pi/4];
    
    out =  - damp * dq - spring * (q-q_d);

== matlab function check_other_Potential/Liu1/MATLAB Function6 ==
  data: M input; E output; y input; spring input; q_d input
function E = energy(M,y,spring, q_d)
    q = y(1:3);
    dq = y(4:6);
    

    E = 0.5 * (dq' * M * dq) + 0.5 * (q-q_d)' *spring* (q-q_d);

== matlab function check_other_Potential/Liu1/MATLAB Function7 ==
  data: M_dot input; out_1 output; S input; q input; out_2 output


function [out_1, out_2] = M_dot_coriolis_check(M_dot,S, q)
    dq = reshape(q(4:6),[3,1]);
    
    q1 = q(1);
    q2 = q(2);
    q3 = q(3);
    dq1 = q(4);
    dq2 = q(5);
    dq3 = q(6);

    check = M_dot - 2 * S;


    out_1 = dq' * check * dq;


    M_dot_formula =   [        - dq2*(sin(q2 + q3) + 3*sin(q2)) - dq3*(sin(q2 + q3) + sin(q3)), - dq3*(sin(q2 + q3)/2 + sin(q3)) - dq2*(sin(q2 + q3)/2 + (3*sin(q2))/2), - (dq2*sin(q2 + q3))/2 - dq3*(sin(q2 + q3)/2 + sin(q3)/2);
- dq3*(sin(q2 + q3)/2 + sin(q3)) - dq2*(sin(q2 + q3)/2 + (3*sin(q2))/2),                                                            -dq3*sin(q3),                                          -(dq3*sin(q3))/2;
              - (dq2*sin(q2 + q3))/2 - dq3*(sin(q2 + q3)/2 + sin(q3)/2),                                                        -(dq3*sin(q3))/2,                                                         0];
 

    
    out_2 = dq' * (M_dot_formula - 2 * S) * dq;
end

== matlab function check_other_Potential/Liu2/MATLAB Function ==
  data: u_des input; damp input; M input; y input; y output; C input; H_dot output; u_sc input; safety input; norm_u_tot output
function [y,H_dot,norm_u_tot]= dynamics(u_des, damp , M,y, C, u_sc, safety)
    
    q = reshape(y(1:3),[3,1]);
    dq = reshape(y(4:6),[3,1]);



    [~, p] = chol(M);
    decision = (p == 0);

    assert(decision, 'Inertia matrix is not positive definite');
    
    u_tot = u_des + safety * u_sc;
    norm_u_tot=norm(u_tot);
    ddq = inv(M) * (u_tot - C * dq ); % + u_sc

    H_dot = - dq' * damp * dq;

    y = [dq; ddq];

== matlab function check_other_Potential/Liu2/MATLAB Function1 ==
  data: y input; M output
function M = inertia_M(y)

    q1 = y(1);
    q2 = y(2);
    q3 = y(3);

    M  = [        cos(q2 + q3) + 3*cos(q2) + cos(q3) + 4, cos(q2 + q3)/2 + (3*cos(q2))/2 + cos(q3) + 5/3, cos(q2 + q3)/2 + cos(q3)/2 + 1/3;
cos(q2 + q3)/2 + (3*cos(q2))/2 + cos(q3) + 5/3,                                  cos(q3) + 5/3,                  cos(q3)/2 + 1/3;
              cos(q2 + q3)/2 + cos(q3)/2 + 1/3,                                cos(q3)/2 + 1/3,                              1/3];

    assert(isequal(M, M'),'error')

== matlab function check_other_Potential/Liu2/MATLAB Function2 ==
  data: y input; C output
function C = coriolis(y)

    q1 = y(1);
    q2 = y(2);
    q3 = y(3);
    dq1 = y(4);
    dq2 = y(5);
    dq3 = y(6);


    C = [- dq2*(sin(q2 + q3)/2 + (3*sin(q2))/2) - dq3*(sin(q2 + q3)/2 + sin(q3)/2), - dq1*(sin(q2 + q3)/2 + (3*sin(q2))/2) - dq2*(sin(q2 + q3)/2 + (3*sin(q2))/2) - dq3*(sin(q2 + q3)/2 + sin(q3)/2), - dq1*(sin(q2 + q3)/2 + sin(q3)/2) - dq2*(sin(q2 + q3)/2 + sin(q3)/2) - dq3*(sin(q2 + q3)/2 + sin(q3)/2);
                dq1*(sin(q2 + q3)/2 + (3*sin(q2))/2) - (dq3*sin(q3))/2,                                                                                                 -(dq3*sin(q3))/2,                                                    - (dq1*sin(q3))/2 - (dq2*sin(q3))/2 - (dq3*sin(q3))/2;
                       dq1*(sin(q2 + q3)/2 + sin(q3)/2) + (dq2*sin(q3))/2,                                                                                (dq1*sin(q3))/2 + (dq2*sin(q3))/2,                                                                                                        0];

== matlab function check_other_Potential/Liu2/MATLAB Function3 ==
  data: C input; y input; cbf_control output; M input; h input; dh_dq input; hessian input; u_des input; psi output; psi_mod output; before_dot output; H_dot output; damp input; hessian_term output; cbf output; cbf_dot output; alpha input; after_dot output; dissipated output

function [cbf_control, psi, psi_mod,before_dot, H_dot, hessian_term, cbf, cbf_dot, after_dot, dissipated]= CBF(C, y, M, h, dh_dq, hessian, u_des, damp, alpha)
% Define numerical values for the parameters
    xc = 2.5;
    yc = 2;
    r = 1;
    gamma = 2;

    
    m1 = 1;
    m2 = 1;
    m3 = 1;
    
    l1 = 1;
    l2 = 1;
    l3 = 1;
    
    q = reshape(y(1:3),[3,1]);
    dq = reshape(y(4:6),[3,1]);
    dh_dq = reshape(dh_dq,[1,3]);

    LIU = 0;

    M_inv = inv(M);

    before_dot = dh_dq * dq;
    after_dot = dh_dq * M_inv * dq;

    d = eig(M_inv);
    tol = 10^(-5);
    check = all(abs(M_inv - M_inv') < tol, 'all');
    assert(check,'error')
    % assert(isequal(M_inv, M_inv'),'error')

    assert(all(d>0),'error_m_inv')

    active = 0;

    if LIU == 1

    
        cbf = alpha * h + dh_dq * dq;
        lg_h = zeros(1,3);
        cbf_dot_prior = alpha .* dh_dq * dq + dq' * hessian * dq + dh_dq * (M_inv* (-C * dq + u_des));
        psi = cbf_dot_prior + gamma .* cbf;
        if psi<0
            lg_h = dh_dq * M_inv;
            
            cbf_control =  - lg_h' /(lg_h * lg_h')  .* psi;
            active = 1;
        else
            cbf_control = zeros(3,1);

        end
        cbf_dot = alpha .* dh_dq * dq + dq' * hessian * dq + dh_dq * M_inv* (-C * dq + u_des+ cbf_control);
        psi_mod = cbf_dot + gamma .* cbf;

        H_dot = dq' * cbf_control - dq' * damp * dq;
        
        dissipated= - dq' * damp * dq;

        hessian_term = dq' * hessian * dq;
        
    
    else
        KE = 0.5 * dq' * M * dq;
        cbf = alpha * h - KE;
        lg_h = zeros(1,3);
        cbf_dot_prior = alpha .* dh_dq * dq - dq' * M_inv * u_des;
        psi = cbf_dot_prior + gamma .* cbf;
        if psi<0
            lg_h = -dq';
            cbf_control =  dq /(dq'*dq)  .* psi;
        else
            cbf_control = zeros(3,1);
        end
        cbf_dot =  alpha .* dh_dq * dq - dq' * M_inv * (u_des+cbf_control) ;
        psi_mod = cbf_dot + gamma .* cbf;

        H_dot = dq' * cbf_control - dq' * damp * dq;


        dissipated= - dq' * damp * dq;

        hessian_term = 0;
 
        
    end
    
end

== matlab function check_other_Potential/Liu2/MATLAB Function4 ==
  data: y input; h output; dh_dq output; hessian_sym output
function [h, dh_dq, hessian_sym] = obstacle(y)
    % Define numerical values for the parameters
    xc = 2.5;
    yc = 2;
    r = 1;

    l1 = 1;
    l2 = 1;
    l3 = 1;
    
    % Compute the end-effector position using forward kinematics
    q1 = y(1);
    q2 = y(2);
    q3 = y(3);
    
    x_ee = l1 * cos(q1) + l2 * cos(q1 + q2) + l3 * cos(q1 + q2 + q3);
    y_ee = l1 * sin(q1) + l2 * sin(q1 + q2) + l3 * sin(q1 + q2 + q3);
    
    % Compute the control barrier function h
    h = (xc - x_ee)^2 + (yc - y_ee)^2 - r^2;
    
    % Define the expressions for dh_dq and hessian_sym
    dh_dq = [2*(cos(q1 + q2 + q3) + cos(q1 + q2) + cos(q1))*(sin(q1 + q2 + q3) + sin(q1 + q2) + sin(q1) - 2) - 2*(sin(q1 + q2 + q3) + sin(q1 + q2) + sin(q1))*(cos(q1 + q2 + q3) + cos(q1 + q2) + cos(q1) - 5/2), 2*(cos(q1 + q2 + q3) + cos(q1 + q2))*(sin(q1 + q2 + q3) + sin(q1 + q2) + sin(q1) - 2) - 2*(sin(q1 + q2 + q3) + sin(q1 + q2))*(cos(q1 + q2 + q3) + cos(q1 + q2) + cos(q1) - 5/2), 2*cos(q1 + q2 + q3)*(sin(q1 + q2 + q3) + sin(q1 + q2) + sin(q1) - 2) - 2*sin(q1 + q2 + q3)*(cos(q1 + q2 + q3) + cos(q1 + q2) + cos(q1) - 5/2)];


    hessian_sym = [                                              2*(cos(q1 + q2 + q3) + cos(q1 + q2) + cos(q1))^2 - 2*(cos(q1 + q2 + q3) + cos(q1 + q2) + cos(q1))*(cos(q1 + q2 + q3) + cos(q1 + q2) + cos(q1) - 5/2) + 2*(sin(q1 + q2 + q3) + sin(q1 + q2) + sin(q1))^2 - 2*(sin(q1 + q2 + q3) + sin(q1 + q2) + sin(q1))*(sin(q1 + q2 + q3) + sin(q1 + q2) + sin(q1) - 2), 2*(cos(q1 + q2 + q3) + cos(q1 + q2))*(cos(q1 + q2 + q3) + cos(q1 + q2) + cos(q1)) - 2*(cos(q1 + q2 + q3) + cos(q1 + q2))*(cos(q1 + q2 + q3) + cos(q1 + q2) + cos(q1) - 5/2) + 2*(sin(q1 + q2 + q3) + sin(q1 + q2))*(sin(q1 + q2 + q3) + sin(q1 + q2) + sin(q1)) - 2*(sin(q1 + q2 + q3) + sin(q1 + q2))*(sin(q1 + q2 + q3) + sin(q1 + q2) + sin(q1) - 2), 2*cos(q1 + q2 + q3)*(cos(q1 + q2 + q3) + cos(q1 + q2) + cos(q1)) - 2*cos(q1 + q2 + q3)*(cos(q1 + q2 + q3) + cos(q1 + q2) + cos(q1) - 5/2) + 2*sin(q1 + q2 + q3)*(sin(q1 + q2 + q3) + sin(q1 + q2) + sin(q1)) - 2*sin(q1 + q2 + q3)*(sin(q1 + q2 + q3) + sin(q1 + q2) + sin(q1) - 2);
        2*(cos(q1 + q2 + q3) + cos(q1 + q2))*(cos(q1 + q2 + q3) + cos(q1 + q2) + cos(q1)) - 2*(cos(q1 + q2 + q3) + cos(q1 + q2))*(cos(q1 + q2 + q3) + cos(q1 + q2) + cos(q1) - 5/2) + 2*(sin(q1 + q2 + q3) + sin(q1 + q2))*(sin(q1 + q2 + q3) + sin(q1 + q2) + sin(q1)) - 2*(sin(q1 + q2 + q3) + sin(q1 + q2))*(sin(q1 + q2 + q3) + sin(q1 + q2) + sin(q1) - 2),                                                                                       2*(cos(q1 + q2 + q3) + cos(q1 + q2))^2 - 2*(cos(q1 + q2 + q3) + cos(q1 + q2))*(cos(q1 + q2 + q3) + cos(q1 + q2) + cos(q1) - 5/2) + 2*(sin(q1 + q2 + q3) + sin(q1 + q2))^2 - 2*(sin(q1 + q2 + q3) + sin(q1 + q2))*(sin(q1 + q2 + q3) + sin(q1 + q2) + sin(q1) - 2),                     2*cos(q1 + q2 + q3)*(cos(q1 + q2 + q3) + cos(q1 + q2)) - 2*cos(q1 + q2 + q3)*(cos(q1 + q2 + q3) + cos(q1 + q2) + cos(q1) - 5/2) - 2*sin(q1 + q2 + q3)*(sin(q1 + q2 + q3) + sin(q1 + q2) + sin(q1) - 2) + 2*sin(q1 + q2 + q3)*(sin(q1 + q2 + q3) + sin(q1 + q2));
                                                                            2*cos(q1 + q2 + q3)*(cos(q1 + q2 + q3) + cos(q1 + q2) + cos(q1)) - 2*cos(q1 + q2 + q3)*(cos(q1 + q2 + q3) + cos(q1 + q2) + cos(q1) - 5/2) + 2*sin(q1 + q2 + q3)*(sin(q1 + q2 + q3) + sin(q1 + q2) + sin(q1)) - 2*sin(q1 + q2 + q3)*(sin(q1 + q2 + q3) + sin(q1 + q2) + sin(q1) - 2),                                                                                         2*cos(q1 + q2 + q3)*(cos(q1 + q2 + q3) + cos(q1 + q2)) - 2*cos(q1 + q2 + q3)*(cos(q1 + q2 + q3) + cos(q1 + q2) + cos(q1) - 5/2) - 2*sin(q1 + q2 + q3)*(sin(q1 + q2 + q3) + sin(q1 + q2) + sin(q1) - 2) + 2*sin(q1 + q2 + q3)*(sin(q1 + q2 + q3) + sin(q1 + q2)),                                                                                       2*cos(q1 + q2 + q3)^2 - 2*cos(q1 + q2 + q3)*(cos(q1 + q2 + q3) + cos(q1 + q2) + cos(q1) - 5/2) + 2*sin(q1 + q2 + q3)^2 - 2*sin(q1 + q2 + q3)*(sin(q1 + q2 + q3) + sin(q1 + q2) + sin(q1) - 2)];
     

    % d = eig(hessian_sym)
    % isposdef = all(d >= 0);
    % 
    % assert(isposdef, 'error hessian');
end

== matlab function check_other_Potential/Liu2/MATLAB Function5 ==
  data: q_d output; y input; spring input; out output; damp input
function [q_d, out] = u_des(y, spring, damp)


    q = reshape(y(1:3),[3,1]);
    dq = reshape(y(4:6),[3,1]);

    q_d = [pi; 0; pi/4];
    
    out =  - damp * dq - spring * (q-q_d);

== matlab function check_other_Potential/Liu/MATLAB Function1 ==
  data: y input; M output
function M = inertia_M(y)

    q1 = y(1);
    q2 = y(2);
    q3 = y(3);

    M  = [        cos(q2 + q3) + 3*cos(q2) + cos(q3) + 4, cos(q2 + q3)/2 + (3*cos(q2))/2 + cos(q3) + 5/3, cos(q2 + q3)/2 + cos(q3)/2 + 1/3;
cos(q2 + q3)/2 + (3*cos(q2))/2 + cos(q3) + 5/3,                                  cos(q3) + 5/3,                  cos(q3)/2 + 1/3;
              cos(q2 + q3)/2 + cos(q3)/2 + 1/3,                                cos(q3)/2 + 1/3,                              1/3];

    assert(isequal(M, M'),'error')

== matlab function check_other_Potential/Liu2/MATLAB Function6 ==
  data: M input; E output; y input; spring input; q_d input
function E = energy(M,y,spring, q_d)
    q = y(1:3);
    dq = y(4:6);
    

    E = 0.5 * (dq' * M * dq) + 0.5 * (q-q_d)' *spring* (q-q_d);

== matlab function check_other_Potential/Liu2/MATLAB Function7 ==
  data: M_dot input; out_1 output; S input; q input; out_2 output


function [out_1, out_2] = M_dot_coriolis_check(M_dot,S, q)
    dq = reshape(q(4:6),[3,1]);
    
    q1 = q(1);
    q2 = q(2);
    q3 = q(3);
    dq1 = q(4);
    dq2 = q(5);
    dq3 = q(6);

    check = M_dot - 2 * S;


    out_1 = dq' * check * dq;


    M_dot_formula =   [        - dq2*(sin(q2 + q3) + 3*sin(q2)) - dq3*(sin(q2 + q3) + sin(q3)), - dq3*(sin(q2 + q3)/2 + sin(q3)) - dq2*(sin(q2 + q3)/2 + (3*sin(q2))/2), - (dq2*sin(q2 + q3))/2 - dq3*(sin(q2 + q3)/2 + sin(q3)/2);
- dq3*(sin(q2 + q3)/2 + sin(q3)) - dq2*(sin(q2 + q3)/2 + (3*sin(q2))/2),                                                            -dq3*sin(q3),                                          -(dq3*sin(q3))/2;
              - (dq2*sin(q2 + q3))/2 - dq3*(sin(q2 + q3)/2 + sin(q3)/2),                                                        -(dq3*sin(q3))/2,                                                         0];
 

    
    out_2 = dq' * (M_dot_formula - 2 * S) * dq;
end

== matlab function check_other_Potential/Liu/MATLAB Function ==
  data: u_des input; damp input; M input; y input; y output; C input; H_dot output; u_sc input; safety input; norm_u_tot output
function [y,H_dot,norm_u_tot]= dynamics(u_des, damp , M,y, C, u_sc, safety)
    
    q = reshape(y(1:3),[3,1]);
    dq = reshape(y(4:6),[3,1]);



    [~, p] = chol(M);
    decision = (p == 0);

    assert(decision, 'Inertia matrix is not positive definite');
    
    u_tot = u_des + safety * u_sc;
    norm_u_tot=norm(u_tot);
    ddq = inv(M) * (u_tot - C * dq ); % + u_sc

    H_dot = - dq' * damp * dq;

    y = [dq; ddq];

== matlab function check_other_Potential/Liu/MATLAB Function2 ==
  data: y input; C output
function C = coriolis(y)

    q1 = y(1);
    q2 = y(2);
    q3 = y(3);
    dq1 = y(4);
    dq2 = y(5);
    dq3 = y(6);


    C = [- dq2*(sin(q2 + q3)/2 + (3*sin(q2))/2) - dq3*(sin(q2 + q3)/2 + sin(q3)/2), - dq1*(sin(q2 + q3)/2 + (3*sin(q2))/2) - dq2*(sin(q2 + q3)/2 + (3*sin(q2))/2) - dq3*(sin(q2 + q3)/2 + sin(q3)/2), - dq1*(sin(q2 + q3)/2 + sin(q3)/2) - dq2*(sin(q2 + q3)/2 + sin(q3)/2) - dq3*(sin(q2 + q3)/2 + sin(q3)/2);
                dq1*(sin(q2 + q3)/2 + (3*sin(q2))/2) - (dq3*sin(q3))/2,                                                                                                 -(dq3*sin(q3))/2,                                                    - (dq1*sin(q3))/2 - (dq2*sin(q3))/2 - (dq3*sin(q3))/2;
                       dq1*(sin(q2 + q3)/2 + sin(q3)/2) + (dq2*sin(q3))/2,                                                                                (dq1*sin(q3))/2 + (dq2*sin(q3))/2,                                                                                                        0];

== matlab function check_other_Potential/Liu/MATLAB Function3 ==
  data: C input; y input; cbf_control output; M input; h input; dh_dq input; hessian input; u_des input; psi output; psi_mod output; before_dot output; H_dot output; damp input; hessian_term output; cbf output; cbf_dot output; alpha input; after_dot output; dissipated output

function [cbf_control, psi, psi_mod,before_dot, H_dot, hessian_term, cbf, cbf_dot, after_dot, dissipated]= CBF(C, y, M, h, dh_dq, hessian, u_des, damp, alpha)
% Define numerical values for the parameters
    xc = 2.5;
    yc = 2;
    r = 1;
    gamma = 2;

    
    m1 = 1;
    m2 = 1;
    m3 = 1;
    
    l1 = 1;
    l2 = 1;
    l3 = 1;
    
    q = reshape(y(1:3),[3,1]);
    dq = reshape(y(4:6),[3,1]);
    dh_dq = reshape(dh_dq,[1,3]);

    LIU = 1;

    M_inv = inv(M);

    before_dot = dh_dq * dq;
    after_dot = dh_dq * M_inv * dq;

    d = eig(M_inv);
    tol = 10^(-5);
    check = all(abs(M_inv - M_inv') < tol, 'all');
    assert(check,'error')
    % assert(isequal(M_inv, M_inv'),'error')

    assert(all(d>0),'error_m_inv')

    active = 0;

    if LIU == 1

    
        cbf = alpha * h + dh_dq * dq;
        lg_h = zeros(1,3);
        cbf_dot_prior = alpha .* dh_dq * dq + dq' * hessian * dq + dh_dq * (M_inv* (-C * dq + u_des));
        psi = cbf_dot_prior + gamma .* cbf;
        if psi<0
            lg_h = dh_dq * M_inv;
            
            cbf_control =  - lg_h' /(lg_h * lg_h')  .* psi;
            active = 1;
        else
            cbf_control = zeros(3,1);

        end
        cbf_dot = alpha .* dh_dq * dq + dq' * hessian * dq + dh_dq * M_inv* (-C * dq + u_des+ cbf_control);
        psi_mod = cbf_dot + gamma .* cbf;

        H_dot = dq' * cbf_control - dq' * damp * dq;
        
        dissipated= - dq' * damp * dq;

        hessian_term = dq' * hessian * dq;
        
    
    else
        KE = 0.5 * dq' * M * dq;
        cbf = alpha * h - KE;
        lg_h = zeros(1,3);
        cbf_dot_prior = alpha .* dh_dq * dq - dq' * M_inv * u_des;
        psi = cbf_dot_prior + gamma .* cbf;
        if psi<0
            lg_h = -dq';
            cbf_control =  dq /(dq'*dq)  .* psi;
        else
            cbf_control = zeros(3,1);
        end
        cbf_dot =  alpha .* dh_dq * dq - dq' * M_inv * (u_des+cbf_control) ;
        psi_mod = cbf_dot + gamma .* cbf;

        H_dot = dq' * cbf_control - dq' * damp * dq;


        hessian_term = 0;
 
        
    end
    
end

== matlab function check_other_Potential/Liu/MATLAB Function4 ==
  data: y input; h output; dh_dq output; hessian_sym output
function [h, dh_dq, hessian_sym] = obstacle(y)
    % Define numerical values for the parameters
    xc = 2.5;
    yc = 2;
    r = 1;

    l1 = 1;
    l2 = 1;
    l3 = 1;
    
    % Compute the end-effector position using forward kinematics
    q1 = y(1);
    q2 = y(2);
    q3 = y(3);
    
    x_ee = l1 * cos(q1) + l2 * cos(q1 + q2) + l3 * cos(q1 + q2 + q3);
    y_ee = l1 * sin(q1) + l2 * sin(q1 + q2) + l3 * sin(q1 + q2 + q3);
    
    % Compute the control barrier function h
    h = (xc - x_ee)^2 + (yc - y_ee)^2 - r^2;
    
    % Define the expressions for dh_dq and hessian_sym
    dh_dq = [2*(cos(q1 + q2 + q3) + cos(q1 + q2) + cos(q1))*(sin(q1 + q2 + q3) + sin(q1 + q2) + sin(q1) - 2) - 2*(sin(q1 + q2 + q3) + sin(q1 + q2) + sin(q1))*(cos(q1 + q2 + q3) + cos(q1 + q2) + cos(q1) - 5/2), 2*(cos(q1 + q2 + q3) + cos(q1 + q2))*(sin(q1 + q2 + q3) + sin(q1 + q2) + sin(q1) - 2) - 2*(sin(q1 + q2 + q3) + sin(q1 + q2))*(cos(q1 + q2 + q3) + cos(q1 + q2) + cos(q1) - 5/2), 2*cos(q1 + q2 + q3)*(sin(q1 + q2 + q3) + sin(q1 + q2) + sin(q1) - 2) - 2*sin(q1 + q2 + q3)*(cos(q1 + q2 + q3) + cos(q1 + q2) + cos(q1) - 5/2)];


    hessian_sym = [                                              2*(cos(q1 + q2 + q3) + cos(q1 + q2) + cos(q1))^2 - 2*(cos(q1 + q2 + q3) + cos(q1 + q2) + cos(q1))*(cos(q1 + q2 + q3) + cos(q1 + q2) + cos(q1) - 5/2) + 2*(sin(q1 + q2 + q3) + sin(q1 + q2) + sin(q1))^2 - 2*(sin(q1 + q2 + q3) + sin(q1 + q2) + sin(q1))*(sin(q1 + q2 + q3) + sin(q1 + q2) + sin(q1) - 2), 2*(cos(q1 + q2 + q3) + cos(q1 + q2))*(cos(q1 + q2 + q3) + cos(q1 + q2) + cos(q1)) - 2*(cos(q1 + q2 + q3) + cos(q1 + q2))*(cos(q1 + q2 + q3) + cos(q1 + q2) + cos(q1) - 5/2) + 2*(sin(q1 + q2 + q3) + sin(q1 + q2))*(sin(q1 + q2 + q3) + sin(q1 + q2) + sin(q1)) - 2*(sin(q1 + q2 + q3) + sin(q1 + q2))*(sin(q1 + q2 + q3) + sin(q1 + q2) + sin(q1) - 2), 2*cos(q1 + q2 + q3)*(cos(q1 + q2 + q3) + cos(q1 + q2) + cos(q1)) - 2*cos(q1 + q2 + q3)*(cos(q1 + q2 + q3) + cos(q1 + q2) + cos(q1) - 5/2) + 2*sin(q1 + q2 + q3)*(sin(q1 + q2 + q3) + sin(q1 + q2) + sin(q1)) - 2*sin(q1 + q2 + q3)*(sin(q1 + q2 + q3) + sin(q1 + q2) + sin(q1) - 2);
        2*(cos(q1 + q2 + q3) + cos(q1 + q2))*(cos(q1 + q2 + q3) + cos(q1 + q2) + cos(q1)) - 2*(cos(q1 + q2 + q3) + cos(q1 + q2))*(cos(q1 + q2 + q3) + cos(q1 + q2) + cos(q1) - 5/2) + 2*(sin(q1 + q2 + q3) + sin(q1 + q2))*(sin(q1 + q2 + q3) + sin(q1 + q2) + sin(q1)) - 2*(sin(q1 + q2 + q3) + sin(q1 + q2))*(sin(q1 + q2 + q3) + sin(q1 + q2) + sin(q1) - 2),                                                                                       2*(cos(q1 + q2 + q3) + cos(q1 + q2))^2 - 2*(cos(q1 + q2 + q3) + cos(q1 + q2))*(cos(q1 + q2 + q3) + cos(q1 + q2) + cos(q1) - 5/2) + 2*(sin(q1 + q2 + q3) + sin(q1 + q2))^2 - 2*(sin(q1 + q2 + q3) + sin(q1 + q2))*(sin(q1 + q2 + q3) + sin(q1 + q2) + sin(q1) - 2),                     2*cos(q1 + q2 + q3)*(cos(q1 + q2 + q3) + cos(q1 + q2)) - 2*cos(q1 + q2 + q3)*(cos(q1 + q2 + q3) + cos(q1 + q2) + cos(q1) - 5/2) - 2*sin(q1 + q2 + q3)*(sin(q1 + q2 + q3) + sin(q1 + q2) + sin(q1) - 2) + 2*sin(q1 + q2 + q3)*(sin(q1 + q2 + q3) + sin(q1 + q2));
                                                                            2*cos(q1 + q2 + q3)*(cos(q1 + q2 + q3) + cos(q1 + q2) + cos(q1)) - 2*cos(q1 + q2 + q3)*(cos(q1 + q2 + q3) + cos(q1 + q2) + cos(q1) - 5/2) + 2*sin(q1 + q2 + q3)*(sin(q1 + q2 + q3) + sin(q1 + q2) + sin(q1)) - 2*sin(q1 + q2 + q3)*(sin(q1 + q2 + q3) + sin(q1 + q2) + sin(q1) - 2),                                                                                         2*cos(q1 + q2 + q3)*(cos(q1 + q2 + q3) + cos(q1 + q2)) - 2*cos(q1 + q2 + q3)*(cos(q1 + q2 + q3) + cos(q1 + q2) + cos(q1) - 5/2) - 2*sin(q1 + q2 + q3)*(sin(q1 + q2 + q3) + sin(q1 + q2) + sin(q1) - 2) + 2*sin(q1 + q2 + q3)*(sin(q1 + q2 + q3) + sin(q1 + q2)),                                                                                       2*cos(q1 + q2 + q3)^2 - 2*cos(q1 + q2 + q3)*(cos(q1 + q2 + q3) + cos(q1 + q2) + cos(q1) - 5/2) + 2*sin(q1 + q2 + q3)^2 - 2*sin(q1 + q2 + q3)*(sin(q1 + q2 + q3) + sin(q1 + q2) + sin(q1) - 2)];
     

    % d = eig(hessian_sym)
    % isposdef = all(d >= 0);
    % 
    % assert(isposdef, 'error hessian');
end

== matlab function check_other_Potential/Liu/MATLAB Function5 ==
  data: q_d output; y input; spring input; out output; damp input
function [q_d, out] = u_des(y, spring, damp)


    q = reshape(y(1:3),[3,1]);
    dq = reshape(y(4:6),[3,1]);

    q_d = [pi; 0; pi/4];
    
    out =  - damp * dq - spring * (q-q_d);
